simulink model "Perception"  (R2024b)
settings: Solver=FixedStepAuto  StartTime=0.0  StopTime=10.0  RelTol=1e-3
undefined symbols (not defined in the file or in its folder): gray
libraries: visiongeotforms x1
settings Model: Creator=csamak  LastModifiedBy=csamak
settings OptimizationCC: ZeroExternalMemoryAtStartup=off  ZeroInternalMemoryAtStartup=off  InitFltsAndDblsToZero=on
settings HardwareCC: ProdLongLongMode=on  TargetLongLongMode=on
settings RTWCC: TargetLang=C++  GenerateGPUCode=CUDA
settings GRTTargetCC: TargetLangStandard=C++11 (ISO)  CodeInterfacePackaging=C++ class

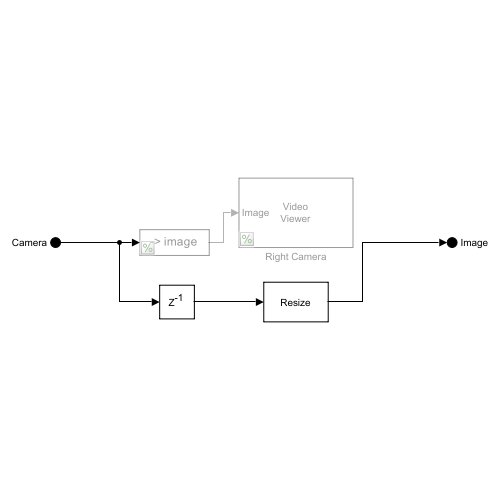
[thumbnail: Simulink's stored preview of the top-level diagram]
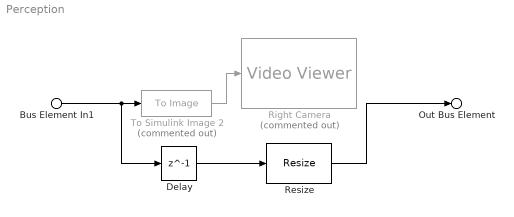
== system Perception ==
  Bus Element In1 : Inport  PortName=Camera
  Delay : Delay  DelayLength=1
  Resize : visiongeotforms/Resize  specify=Number of output rows and columns  rfactor=[200 150]  outCols=25  outRows=25  outRowsCols=[360 640]  interp_method=Bilinear  antialias=on  useROI=off  roiFlag=off  roundingMode=Nearest  overflowMode=on  prodOutputMode=Binary point scaling  prodOutputWordLength=32  prodOutputFracLength=10
  Right Camera : VideoViewer  Commented=on  colormapValue=gray(256)  FigPos=[2.33333333333333 406.666666666667 418 304]
  To Simulink Image 2 : ToImage  Commented=on
  Out Bus Element : Outport  PortName=Image
  wires:
  Delay/1 -> Resize/1
  To Simulink Image 2/1 -> Right Camera/1
  Bus Element In1/1 -> Delay/1, To Simulink Image 2/1
  Resize/1 -> Out Bus Element/1
